simulink model "Filter_Fixed"  (R2017b)
settings: Solver=FixedStepDiscrete  StartTime=0.0  StopTime=400  RelTol=1e-3
undefined symbols (not defined in the file or in its folder): designMultirateFIR
libraries: dspmlti4 x1
(part 2 of 3)

== system Filter_Fixed/HighpassH/Resonator116 ==
  In1 : Inport
  Delay : Delay  DelayLength=1
  Gain : Gain  Gain=-0.67188-0.74066i  OutDataTypeStr=fixdt(1,24,23)
  GainH : Gain  Gain=0.39229-0.91984i  OutDataTypeStr=fixdt(1,24,23)
  Sum1 : Sum  Inputs=|++
  Out1 : Outport
  wires:
  In1/1 -> Sum1/1
  GainH/1 -> Out1/1
  Gain/1 -> Sum1/2
  Delay/1 -> Gain/1
  Sum1/1 -> Delay/1, GainH/1

== system Filter_Fixed/HighpassH/Resonator117 ==
  In1 : Inport
  Delay : Delay  DelayLength=1
  Gain : Gain  Gain=-0.65103-0.75905i  OutDataTypeStr=fixdt(1,24,23)
  GainH : Gain  Gain=-0.40504+0.9143i  OutDataTypeStr=fixdt(1,24,23)
  Sum1 : Sum  Inputs=|++
  Out1 : Outport
  wires:
  In1/1 -> Sum1/1
  GainH/1 -> Out1/1
  Gain/1 -> Sum1/2
  Delay/1 -> Gain/1
  Sum1/1 -> Delay/1, GainH/1

== system Filter_Fixed/HighpassH/Resonator118 ==
  In1 : Inport
  Delay : Delay  DelayLength=1
  Gain : Gain  Gain=-0.62968-0.77685i  OutDataTypeStr=fixdt(1,24,23)
  GainH : Gain  Gain=0.41771-0.90858i  OutDataTypeStr=fixdt(1,24,23)
  Sum1 : Sum  Inputs=|++
  Out1 : Outport
  wires:
  In1/1 -> Sum1/1
  GainH/1 -> Out1/1
  Gain/1 -> Sum1/2
  Delay/1 -> Gain/1
  Sum1/1 -> Delay/1, GainH/1

== system Filter_Fixed/HighpassH/Resonator119 ==
  In1 : Inport
  Delay : Delay  DelayLength=1
  Gain : Gain  Gain=-0.60784-0.79406i  OutDataTypeStr=fixdt(1,24,23)
  GainH : Gain  Gain=-0.4303+0.90269i  OutDataTypeStr=fixdt(1,24,23)
  Sum1 : Sum  Inputs=|++
  Out1 : Outport
  wires:
  In1/1 -> Sum1/1
  GainH/1 -> Out1/1
  Gain/1 -> Sum1/2
  Delay/1 -> Gain/1
  Sum1/1 -> Delay/1, GainH/1

== system Filter_Fixed/HighpassH/Resonator12 ==
  In1 : Inport
  Delay : Delay  DelayLength=1
  Gain : Gain  Gain=0.46756+0.88396i  OutDataTypeStr=fixdt(1,24,23)
  GainH : Gain  Gain=0.8637+0.50401i  OutDataTypeStr=fixdt(1,24,23)
  Sum1 : Sum  Inputs=|++
  Out1 : Outport
  wires:
  In1/1 -> Sum1/1
  GainH/1 -> Out1/1
  Gain/1 -> Sum1/2
  Delay/1 -> Gain/1
  Sum1/1 -> Delay/1, GainH/1

== system Filter_Fixed/HighpassH/Resonator120 ==
  In1 : Inport
  Delay : Delay  DelayLength=1
  Gain : Gain  Gain=-0.58553-0.81065i  OutDataTypeStr=fixdt(1,24,23)
  GainH : Gain  Gain=0.44281-0.89662i  OutDataTypeStr=fixdt(1,24,23)
  Sum1 : Sum  Inputs=|++
  Out1 : Outport
  wires:
  In1/1 -> Sum1/1
  GainH/1 -> Out1/1
  Gain/1 -> Sum1/2
  Delay/1 -> Gain/1
  Sum1/1 -> Delay/1, GainH/1

== system Filter_Fixed/HighpassH/Resonator121 ==
  In1 : Inport
  Delay : Delay  DelayLength=1
  Gain : Gain  Gain=-0.56277-0.82661i  OutDataTypeStr=fixdt(1,24,23)
  GainH : Gain  Gain=-0.45523+0.89037i  OutDataTypeStr=fixdt(1,24,23)
  Sum1 : Sum  Inputs=|++
  Out1 : Outport
  wires:
  In1/1 -> Sum1/1
  GainH/1 -> Out1/1
  Gain/1 -> Sum1/2
  Delay/1 -> Gain/1
  Sum1/1 -> Delay/1, GainH/1

== system Filter_Fixed/HighpassH/Resonator122 ==
  In1 : Inport
  Delay : Delay  DelayLength=1
  Gain : Gain  Gain=-0.53958-0.84194i  OutDataTypeStr=fixdt(1,24,23)
  GainH : Gain  Gain=0.46756-0.88396i  OutDataTypeStr=fixdt(1,24,23)
  Sum1 : Sum  Inputs=|++
  Out1 : Outport
  wires:
  In1/1 -> Sum1/1
  GainH/1 -> Out1/1
  Gain/1 -> Sum1/2
  Delay/1 -> Gain/1
  Sum1/1 -> Delay/1, GainH/1

== system Filter_Fixed/HighpassH/Resonator123 ==
  In1 : Inport
  Delay : Delay  DelayLength=1
  Gain : Gain  Gain=-0.51596-0.85661i  OutDataTypeStr=fixdt(1,24,23)
  GainH : Gain  Gain=-0.4798+0.87738i  OutDataTypeStr=fixdt(1,24,23)
  Sum1 : Sum  Inputs=|++
  Out1 : Outport
  wires:
  In1/1 -> Sum1/1
  GainH/1 -> Out1/1
  Gain/1 -> Sum1/2
  Delay/1 -> Gain/1
  Sum1/1 -> Delay/1, GainH/1

== system Filter_Fixed/HighpassH/Resonator124 ==
  In1 : Inport
  Delay : Delay  DelayLength=1
  Gain : Gain  Gain=-0.49195-0.87062i  OutDataTypeStr=fixdt(1,24,23)
  GainH : Gain  Gain=0.49195-0.87062i  OutDataTypeStr=fixdt(1,24,23)
  Sum1 : Sum  Inputs=|++
  Out1 : Outport
  wires:
  In1/1 -> Sum1/1
  GainH/1 -> Out1/1
  Gain/1 -> Sum1/2
  Delay/1 -> Gain/1
  Sum1/1 -> Delay/1, GainH/1

== system Filter_Fixed/HighpassH/Resonator125 ==
  In1 : Inport
  Delay : Delay  DelayLength=1
  Gain : Gain  Gain=-0.46756-0.88396i  OutDataTypeStr=fixdt(1,24,23)
  GainH : Gain  Gain=-0.50401+0.8637i  OutDataTypeStr=fixdt(1,24,23)
  Sum1 : Sum  Inputs=|++
  Out1 : Outport
  wires:
  In1/1 -> Sum1/1
  GainH/1 -> Out1/1
  Gain/1 -> Sum1/2
  Delay/1 -> Gain/1
  Sum1/1 -> Delay/1, GainH/1

== system Filter_Fixed/HighpassH/Resonator126 ==
  In1 : Inport
  Delay : Delay  DelayLength=1
  Gain : Gain  Gain=-0.44281-0.89662i  OutDataTypeStr=fixdt(1,24,23)
  GainH : Gain  Gain=0.51596-0.85661i  OutDataTypeStr=fixdt(1,24,23)
  Sum1 : Sum  Inputs=|++
  Out1 : Outport
  wires:
  In1/1 -> Sum1/1
  GainH/1 -> Out1/1
  Gain/1 -> Sum1/2
  Delay/1 -> Gain/1
  Sum1/1 -> Delay/1, GainH/1

== system Filter_Fixed/HighpassH/Resonator127 ==
  In1 : Inport
  Delay : Delay  DelayLength=1
  Gain : Gain  Gain=-0.41771-0.90858i  OutDataTypeStr=fixdt(1,24,23)
  GainH : Gain  Gain=-0.52782+0.84936i  OutDataTypeStr=fixdt(1,24,23)
  Sum1 : Sum  Inputs=|++
  Out1 : Outport
  wires:
  In1/1 -> Sum1/1
  GainH/1 -> Out1/1
  Gain/1 -> Sum1/2
  Delay/1 -> Gain/1
  Sum1/1 -> Delay/1, GainH/1

== system Filter_Fixed/HighpassH/Resonator128 ==
  In1 : Inport
  Delay : Delay  DelayLength=1
  Gain : Gain  Gain=-0.39229-0.91984i  OutDataTypeStr=fixdt(1,24,23)
  GainH : Gain  Gain=0.53958-0.84194i  OutDataTypeStr=fixdt(1,24,23)
  Sum1 : Sum  Inputs=|++
  Out1 : Outport
  wires:
  In1/1 -> Sum1/1
  GainH/1 -> Out1/1
  Gain/1 -> Sum1/2
  Delay/1 -> Gain/1
  Sum1/1 -> Delay/1, GainH/1

== system Filter_Fixed/HighpassH/Resonator129 ==
  In1 : Inport
  Delay : Delay  DelayLength=1
  Gain : Gain  Gain=-0.36657-0.93039i  OutDataTypeStr=fixdt(1,24,23)
  GainH : Gain  Gain=-0.55123+0.83435i  OutDataTypeStr=fixdt(1,24,23)
  Sum1 : Sum  Inputs=|++
  Out1 : Outport
  wires:
  In1/1 -> Sum1/1
  GainH/1 -> Out1/1
  Gain/1 -> Sum1/2
  Delay/1 -> Gain/1
  Sum1/1 -> Delay/1, GainH/1

== system Filter_Fixed/HighpassH/Resonator13 ==
  In1 : Inport
  Delay : Delay  DelayLength=1
  Gain : Gain  Gain=0.44281+0.89662i  OutDataTypeStr=fixdt(1,24,23)
  GainH : Gain  Gain=-0.85661-0.51596i  OutDataTypeStr=fixdt(1,24,23)
  Sum1 : Sum  Inputs=|++
  Out1 : Outport
  wires:
  In1/1 -> Sum1/1
  GainH/1 -> Out1/1
  Gain/1 -> Sum1/2
  Delay/1 -> Gain/1
  Sum1/1 -> Delay/1, GainH/1

== system Filter_Fixed/HighpassH/Resonator130 ==
  In1 : Inport
  Delay : Delay  DelayLength=1
  Gain : Gain  Gain=-0.34057-0.94022i  OutDataTypeStr=fixdt(1,24,23)
  GainH : Gain  Gain=0.56277-0.82661i  OutDataTypeStr=fixdt(1,24,23)
  Sum1 : Sum  Inputs=|++
  Out1 : Outport
  wires:
  In1/1 -> Sum1/1
  GainH/1 -> Out1/1
  Gain/1 -> Sum1/2
  Delay/1 -> Gain/1
  Sum1/1 -> Delay/1, GainH/1

== system Filter_Fixed/HighpassH/Resonator131 ==
  In1 : Inport
  Delay : Delay  DelayLength=1
  Gain : Gain  Gain=-0.3143-0.94932i  OutDataTypeStr=fixdt(1,24,23)
  GainH : Gain  Gain=-0.57421+0.81871i  OutDataTypeStr=fixdt(1,24,23)
  Sum1 : Sum  Inputs=|++
  Out1 : Outport
  wires:
  In1/1 -> Sum1/1
  GainH/1 -> Out1/1
  Gain/1 -> Sum1/2
  Delay/1 -> Gain/1
  Sum1/1 -> Delay/1, GainH/1

== system Filter_Fixed/HighpassH/Resonator132 ==
  In1 : Inport
  Delay : Delay  DelayLength=1
  Gain : Gain  Gain=-0.28779-0.95769i  OutDataTypeStr=fixdt(1,24,23)
  GainH : Gain  Gain=0.58553-0.81065i  OutDataTypeStr=fixdt(1,24,23)
  Sum1 : Sum  Inputs=|++
  Out1 : Outport
  wires:
  In1/1 -> Sum1/1
  GainH/1 -> Out1/1
  Gain/1 -> Sum1/2
  Delay/1 -> Gain/1
  Sum1/1 -> Delay/1, GainH/1

== system Filter_Fixed/HighpassH/Resonator133 ==
  In1 : Inport
  Delay : Delay  DelayLength=1
  Gain : Gain  Gain=-0.26106-0.96532i  OutDataTypeStr=fixdt(1,24,23)
  GainH : Gain  Gain=-0.59675+0.80243i  OutDataTypeStr=fixdt(1,24,23)
  Sum1 : Sum  Inputs=|++
  Out1 : Outport
  wires:
  In1/1 -> Sum1/1
  GainH/1 -> Out1/1
  Gain/1 -> Sum1/2
  Delay/1 -> Gain/1
  Sum1/1 -> Delay/1, GainH/1

== system Filter_Fixed/HighpassH/Resonator134 ==
  In1 : Inport
  Delay : Delay  DelayLength=1
  Gain : Gain  Gain=-0.23412-0.97221i  OutDataTypeStr=fixdt(1,24,23)
  GainH : Gain  Gain=0.60784-0.79406i  OutDataTypeStr=fixdt(1,24,23)
  Sum1 : Sum  Inputs=|++
  Out1 : Outport
  wires:
  In1/1 -> Sum1/1
  GainH/1 -> Out1/1
  Gain/1 -> Sum1/2
  Delay/1 -> Gain/1
  Sum1/1 -> Delay/1, GainH/1

== system Filter_Fixed/HighpassH/Resonator135 ==
  In1 : Inport
  Delay : Delay  DelayLength=1
  Gain : Gain  Gain=-0.20701-0.97834i  OutDataTypeStr=fixdt(1,24,23)
  GainH : Gain  Gain=-0.61882+0.78553i  OutDataTypeStr=fixdt(1,24,23)
  Sum1 : Sum  Inputs=|++
  Out1 : Outport
  wires:
  In1/1 -> Sum1/1
  GainH/1 -> Out1/1
  Gain/1 -> Sum1/2
  Delay/1 -> Gain/1
  Sum1/1 -> Delay/1, GainH/1

== system Filter_Fixed/HighpassH/Resonator136 ==
  In1 : Inport
  Delay : Delay  DelayLength=1
  Gain : Gain  Gain=-0.17973-0.98372i  OutDataTypeStr=fixdt(1,24,23)
  GainH : Gain  Gain=0.62968-0.77685i  OutDataTypeStr=fixdt(1,24,23)
  Sum1 : Sum  Inputs=|++
  Out1 : Outport
  wires:
  In1/1 -> Sum1/1
  GainH/1 -> Out1/1
  Gain/1 -> Sum1/2
  Delay/1 -> Gain/1
  Sum1/1 -> Delay/1, GainH/1

== system Filter_Fixed/HighpassH/Resonator137 ==
  In1 : Inport
  Delay : Delay  DelayLength=1
  Gain : Gain  Gain=-0.15231-0.98833i  OutDataTypeStr=fixdt(1,24,23)
  GainH : Gain  Gain=-0.64042+0.76803i  OutDataTypeStr=fixdt(1,24,23)
  Sum1 : Sum  Inputs=|++
  Out1 : Outport
  wires:
  In1/1 -> Sum1/1
  GainH/1 -> Out1/1
  Gain/1 -> Sum1/2
  Delay/1 -> Gain/1
  Sum1/1 -> Delay/1, GainH/1

== system Filter_Fixed/HighpassH/Resonator138 ==
  In1 : Inport
  Delay : Delay  DelayLength=1
  Gain : Gain  Gain=-0.12478-0.99218i  OutDataTypeStr=fixdt(1,24,23)
  GainH : Gain  Gain=0.65103-0.75905i  OutDataTypeStr=fixdt(1,24,23)
  Sum1 : Sum  Inputs=|++
  Out1 : Outport
  wires:
  In1/1 -> Sum1/1
  GainH/1 -> Out1/1
  Gain/1 -> Sum1/2
  Delay/1 -> Gain/1
  Sum1/1 -> Delay/1, GainH/1

== system Filter_Fixed/HighpassH/Resonator139 ==
  In1 : Inport
  Delay : Delay  DelayLength=1
  Gain : Gain  Gain=-0.097152-0.99527i  OutDataTypeStr=fixdt(1,24,23)
  GainH : Gain  Gain=-0.66152+0.74993i  OutDataTypeStr=fixdt(1,24,23)
  Sum1 : Sum  Inputs=|++
  Out1 : Outport
  wires:
  In1/1 -> Sum1/1
  GainH/1 -> Out1/1
  Gain/1 -> Sum1/2
  Delay/1 -> Gain/1
  Sum1/1 -> Delay/1, GainH/1

== system Filter_Fixed/HighpassH/Resonator14 ==
  In1 : Inport
  Delay : Delay  DelayLength=1
  Gain : Gain  Gain=0.41771+0.90858i  OutDataTypeStr=fixdt(1,24,23)
  GainH : Gain  Gain=0.84936+0.52782i  OutDataTypeStr=fixdt(1,24,23)
  Sum1 : Sum  Inputs=|++
  Out1 : Outport
  wires:
  In1/1 -> Sum1/1
  GainH/1 -> Out1/1
  Gain/1 -> Sum1/2
  Delay/1 -> Gain/1
  Sum1/1 -> Delay/1, GainH/1

== system Filter_Fixed/HighpassH/Resonator140 ==
  In1 : Inport
  Delay : Delay  DelayLength=1
  Gain : Gain  Gain=-0.069448-0.99759i  OutDataTypeStr=fixdt(1,24,23)
  GainH : Gain  Gain=0.67188-0.74066i  OutDataTypeStr=fixdt(1,24,23)
  Sum1 : Sum  Inputs=|++
  Out1 : Outport
  wires:
  In1/1 -> Sum1/1
  GainH/1 -> Out1/1
  Gain/1 -> Sum1/2
  Delay/1 -> Gain/1
  Sum1/1 -> Delay/1, GainH/1

== system Filter_Fixed/HighpassH/Resonator141 ==
  In1 : Inport
  Delay : Delay  DelayLength=1
  Gain : Gain  Gain=-0.04169-0.99913i  OutDataTypeStr=fixdt(1,24,23)
  GainH : Gain  Gain=-0.68211+0.73125i  OutDataTypeStr=fixdt(1,24,23)
  Sum1 : Sum  Inputs=|++
  Out1 : Outport
  wires:
  In1/1 -> Sum1/1
  GainH/1 -> Out1/1
  Gain/1 -> Sum1/2
  Delay/1 -> Gain/1
  Sum1/1 -> Delay/1, GainH/1

== system Filter_Fixed/HighpassH/Resonator142 ==
  In1 : Inport
  Delay : Delay  DelayLength=1
  Gain : Gain  Gain=-0.0139-0.9999i  OutDataTypeStr=fixdt(1,24,23)
  GainH : Gain  Gain=0.69221-0.7217i  OutDataTypeStr=fixdt(1,24,23)
  Sum1 : Sum  Inputs=|++
  Out1 : Outport
  wires:
  In1/1 -> Sum1/1
  GainH/1 -> Out1/1
  Gain/1 -> Sum1/2
  Delay/1 -> Gain/1
  Sum1/1 -> Delay/1, GainH/1

== system Filter_Fixed/HighpassH/Resonator143 ==
  In1 : Inport
  Delay : Delay  DelayLength=1
  Gain : Gain  Gain=0.0139-0.9999i  OutDataTypeStr=fixdt(1,24,23)
  GainH : Gain  Gain=-0.70218+0.712i  OutDataTypeStr=fixdt(1,24,23)
  Sum1 : Sum  Inputs=|++
  Out1 : Outport
  wires:
  In1/1 -> Sum1/1
  GainH/1 -> Out1/1
  Gain/1 -> Sum1/2
  Delay/1 -> Gain/1
  Sum1/1 -> Delay/1, GainH/1

== system Filter_Fixed/HighpassH/Resonator144 ==
  In1 : Inport
  Delay : Delay  DelayLength=1
  Gain : Gain  Gain=0.04169-0.99913i  OutDataTypeStr=fixdt(1,24,23)
  GainH : Gain  Gain=0.712-0.70218i  OutDataTypeStr=fixdt(1,24,23)
  Sum1 : Sum  Inputs=|++
  Out1 : Outport
  wires:
  In1/1 -> Sum1/1
  GainH/1 -> Out1/1
  Gain/1 -> Sum1/2
  Delay/1 -> Gain/1
  Sum1/1 -> Delay/1, GainH/1

== system Filter_Fixed/HighpassH/Resonator145 ==
  In1 : Inport
  Delay : Delay  DelayLength=1
  Gain : Gain  Gain=0.069448-0.99759i  OutDataTypeStr=fixdt(1,24,23)
  GainH : Gain  Gain=-0.7217+0.69221i  OutDataTypeStr=fixdt(1,24,23)
  Sum1 : Sum  Inputs=|++
  Out1 : Outport
  wires:
  In1/1 -> Sum1/1
  GainH/1 -> Out1/1
  Gain/1 -> Sum1/2
  Delay/1 -> Gain/1
  Sum1/1 -> Delay/1, GainH/1

== system Filter_Fixed/HighpassH/Resonator146 ==
  In1 : Inport
  Delay : Delay  DelayLength=1
  Gain : Gain  Gain=0.097152-0.99527i  OutDataTypeStr=fixdt(1,24,23)
  GainH : Gain  Gain=0.73125-0.68211i  OutDataTypeStr=fixdt(1,24,23)
  Sum1 : Sum  Inputs=|++
  Out1 : Outport
  wires:
  In1/1 -> Sum1/1
  GainH/1 -> Out1/1
  Gain/1 -> Sum1/2
  Delay/1 -> Gain/1
  Sum1/1 -> Delay/1, GainH/1

== system Filter_Fixed/HighpassH/Resonator147 ==
  In1 : Inport
  Delay : Delay  DelayLength=1
  Gain : Gain  Gain=0.12478-0.99218i  OutDataTypeStr=fixdt(1,24,23)
  GainH : Gain  Gain=-0.74066+0.67188i  OutDataTypeStr=fixdt(1,24,23)
  Sum1 : Sum  Inputs=|++
  Out1 : Outport
  wires:
  In1/1 -> Sum1/1
  GainH/1 -> Out1/1
  Gain/1 -> Sum1/2
  Delay/1 -> Gain/1
  Sum1/1 -> Delay/1, GainH/1

== system Filter_Fixed/HighpassH/Resonator148 ==
  In1 : Inport
  Delay : Delay  DelayLength=1
  Gain : Gain  Gain=0.15231-0.98833i  OutDataTypeStr=fixdt(1,24,23)
  GainH : Gain  Gain=0.74993-0.66152i  OutDataTypeStr=fixdt(1,24,23)
  Sum1 : Sum  Inputs=|++
  Out1 : Outport
  wires:
  In1/1 -> Sum1/1
  GainH/1 -> Out1/1
  Gain/1 -> Sum1/2
  Delay/1 -> Gain/1
  Sum1/1 -> Delay/1, GainH/1

== system Filter_Fixed/HighpassH/Resonator149 ==
  In1 : Inport
  Delay : Delay  DelayLength=1
  Gain : Gain  Gain=0.17973-0.98372i  OutDataTypeStr=fixdt(1,24,23)
  GainH : Gain  Gain=-0.75905+0.65103i  OutDataTypeStr=fixdt(1,24,23)
  Sum1 : Sum  Inputs=|++
  Out1 : Outport
  wires:
  In1/1 -> Sum1/1
  GainH/1 -> Out1/1
  Gain/1 -> Sum1/2
  Delay/1 -> Gain/1
  Sum1/1 -> Delay/1, GainH/1

== system Filter_Fixed/HighpassH/Resonator15 ==
  In1 : Inport
  Delay : Delay  DelayLength=1
  Gain : Gain  Gain=0.39229+0.91984i  OutDataTypeStr=fixdt(1,24,23)
  GainH : Gain  Gain=-0.84194-0.53958i  OutDataTypeStr=fixdt(1,24,23)
  Sum1 : Sum  Inputs=|++
  Out1 : Outport
  wires:
  In1/1 -> Sum1/1
  GainH/1 -> Out1/1
  Gain/1 -> Sum1/2
  Delay/1 -> Gain/1
  Sum1/1 -> Delay/1, GainH/1

== system Filter_Fixed/HighpassH/Resonator150 ==
  In1 : Inport
  Delay : Delay  DelayLength=1
  Gain : Gain  Gain=0.20701-0.97834i  OutDataTypeStr=fixdt(1,24,23)
  GainH : Gain  Gain=0.76803-0.64042i  OutDataTypeStr=fixdt(1,24,23)
  Sum1 : Sum  Inputs=|++
  Out1 : Outport
  wires:
  In1/1 -> Sum1/1
  GainH/1 -> Out1/1
  Gain/1 -> Sum1/2
  Delay/1 -> Gain/1
  Sum1/1 -> Delay/1, GainH/1

== system Filter_Fixed/HighpassH/Resonator151 ==
  In1 : Inport
  Delay : Delay  DelayLength=1
  Gain : Gain  Gain=0.23412-0.97221i  OutDataTypeStr=fixdt(1,24,23)
  GainH : Gain  Gain=-0.77685+0.62968i  OutDataTypeStr=fixdt(1,24,23)
  Sum1 : Sum  Inputs=|++
  Out1 : Outport
  wires:
  In1/1 -> Sum1/1
  GainH/1 -> Out1/1
  Gain/1 -> Sum1/2
  Delay/1 -> Gain/1
  Sum1/1 -> Delay/1, GainH/1

== system Filter_Fixed/HighpassH/Resonator152 ==
  In1 : Inport
  Delay : Delay  DelayLength=1
  Gain : Gain  Gain=0.26106-0.96532i  OutDataTypeStr=fixdt(1,24,23)
  GainH : Gain  Gain=0.78553-0.61882i  OutDataTypeStr=fixdt(1,24,23)
  Sum1 : Sum  Inputs=|++
  Out1 : Outport
  wires:
  In1/1 -> Sum1/1
  GainH/1 -> Out1/1
  Gain/1 -> Sum1/2
  Delay/1 -> Gain/1
  Sum1/1 -> Delay/1, GainH/1

== system Filter_Fixed/HighpassH/Resonator153 ==
  In1 : Inport
  Delay : Delay  DelayLength=1
  Gain : Gain  Gain=0.28779-0.95769i  OutDataTypeStr=fixdt(1,24,23)
  GainH : Gain  Gain=-0.79406+0.60784i  OutDataTypeStr=fixdt(1,24,23)
  Sum1 : Sum  Inputs=|++
  Out1 : Outport
  wires:
  In1/1 -> Sum1/1
  GainH/1 -> Out1/1
  Gain/1 -> Sum1/2
  Delay/1 -> Gain/1
  Sum1/1 -> Delay/1, GainH/1

== system Filter_Fixed/HighpassH/Resonator154 ==
  In1 : Inport
  Delay : Delay  DelayLength=1
  Gain : Gain  Gain=0.3143-0.94932i  OutDataTypeStr=fixdt(1,24,23)
  GainH : Gain  Gain=0.80243-0.59675i  OutDataTypeStr=fixdt(1,24,23)
  Sum1 : Sum  Inputs=|++
  Out1 : Outport
  wires:
  In1/1 -> Sum1/1
  GainH/1 -> Out1/1
  Gain/1 -> Sum1/2
  Delay/1 -> Gain/1
  Sum1/1 -> Delay/1, GainH/1

== system Filter_Fixed/HighpassH/Resonator155 ==
  In1 : Inport
  Delay : Delay  DelayLength=1
  Gain : Gain  Gain=0.34057-0.94022i  OutDataTypeStr=fixdt(1,24,23)
  GainH : Gain  Gain=-0.81065+0.58553i  OutDataTypeStr=fixdt(1,24,23)
  Sum1 : Sum  Inputs=|++
  Out1 : Outport
  wires:
  In1/1 -> Sum1/1
  GainH/1 -> Out1/1
  Gain/1 -> Sum1/2
  Delay/1 -> Gain/1
  Sum1/1 -> Delay/1, GainH/1

== system Filter_Fixed/HighpassH/Resonator156 ==
  In1 : Inport
  Delay : Delay  DelayLength=1
  Gain : Gain  Gain=0.36657-0.93039i  OutDataTypeStr=fixdt(1,24,23)
  GainH : Gain  Gain=0.81871-0.57421i  OutDataTypeStr=fixdt(1,24,23)
  Sum1 : Sum  Inputs=|++
  Out1 : Outport
  wires:
  In1/1 -> Sum1/1
  GainH/1 -> Out1/1
  Gain/1 -> Sum1/2
  Delay/1 -> Gain/1
  Sum1/1 -> Delay/1, GainH/1

== system Filter_Fixed/HighpassH/Resonator157 ==
  In1 : Inport
  Delay : Delay  DelayLength=1
  Gain : Gain  Gain=0.39229-0.91984i  OutDataTypeStr=fixdt(1,24,23)
  GainH : Gain  Gain=-0.82661+0.56277i  OutDataTypeStr=fixdt(1,24,23)
  Sum1 : Sum  Inputs=|++
  Out1 : Outport
  wires:
  In1/1 -> Sum1/1
  GainH/1 -> Out1/1
  Gain/1 -> Sum1/2
  Delay/1 -> Gain/1
  Sum1/1 -> Delay/1, GainH/1

== system Filter_Fixed/HighpassH/Resonator158 ==
  In1 : Inport
  Delay : Delay  DelayLength=1
  Gain : Gain  Gain=0.41771-0.90858i  OutDataTypeStr=fixdt(1,24,23)
  GainH : Gain  Gain=0.83435-0.55123i  OutDataTypeStr=fixdt(1,24,23)
  Sum1 : Sum  Inputs=|++
  Out1 : Outport
  wires:
  In1/1 -> Sum1/1
  GainH/1 -> Out1/1
  Gain/1 -> Sum1/2
  Delay/1 -> Gain/1
  Sum1/1 -> Delay/1, GainH/1

== system Filter_Fixed/HighpassH/Resonator159 ==
  In1 : Inport
  Delay : Delay  DelayLength=1
  Gain : Gain  Gain=0.44281-0.89662i  OutDataTypeStr=fixdt(1,24,23)
  GainH : Gain  Gain=-0.84194+0.53958i  OutDataTypeStr=fixdt(1,24,23)
  Sum1 : Sum  Inputs=|++
  Out1 : Outport
  wires:
  In1/1 -> Sum1/1
  GainH/1 -> Out1/1
  Gain/1 -> Sum1/2
  Delay/1 -> Gain/1
  Sum1/1 -> Delay/1, GainH/1

== system Filter_Fixed/HighpassH/Resonator16 ==
  In1 : Inport
  Delay : Delay  DelayLength=1
  Gain : Gain  Gain=0.36657+0.93039i  OutDataTypeStr=fixdt(1,24,23)
  GainH : Gain  Gain=0.83435+0.55123i  OutDataTypeStr=fixdt(1,24,23)
  Sum1 : Sum  Inputs=|++
  Out1 : Outport
  wires:
  In1/1 -> Sum1/1
  GainH/1 -> Out1/1
  Gain/1 -> Sum1/2
  Delay/1 -> Gain/1
  Sum1/1 -> Delay/1, GainH/1

== system Filter_Fixed/HighpassH/Resonator160 ==
  In1 : Inport
  Delay : Delay  DelayLength=1
  Gain : Gain  Gain=0.46756-0.88396i  OutDataTypeStr=fixdt(1,24,23)
  GainH : Gain  Gain=0.84936-0.52782i  OutDataTypeStr=fixdt(1,24,23)
  Sum1 : Sum  Inputs=|++
  Out1 : Outport
  wires:
  In1/1 -> Sum1/1
  GainH/1 -> Out1/1
  Gain/1 -> Sum1/2
  Delay/1 -> Gain/1
  Sum1/1 -> Delay/1, GainH/1

== system Filter_Fixed/HighpassH/Resonator161 ==
  In1 : Inport
  Delay : Delay  DelayLength=1
  Gain : Gain  Gain=0.49195-0.87062i  OutDataTypeStr=fixdt(1,24,23)
  GainH : Gain  Gain=-0.85661+0.51596i  OutDataTypeStr=fixdt(1,24,23)
  Sum1 : Sum  Inputs=|++
  Out1 : Outport
  wires:
  In1/1 -> Sum1/1
  GainH/1 -> Out1/1
  Gain/1 -> Sum1/2
  Delay/1 -> Gain/1
  Sum1/1 -> Delay/1, GainH/1

== system Filter_Fixed/HighpassH/Resonator162 ==
  In1 : Inport
  Delay : Delay  DelayLength=1
  Gain : Gain  Gain=0.51596-0.85661i  OutDataTypeStr=fixdt(1,24,23)
  GainH : Gain  Gain=0.8637-0.50401i  OutDataTypeStr=fixdt(1,24,23)
  Sum1 : Sum  Inputs=|++
  Out1 : Outport
  wires:
  In1/1 -> Sum1/1
  GainH/1 -> Out1/1
  Gain/1 -> Sum1/2
  Delay/1 -> Gain/1
  Sum1/1 -> Delay/1, GainH/1

== system Filter_Fixed/HighpassH/Resonator163 ==
  In1 : Inport
  Delay : Delay  DelayLength=1
  Gain : Gain  Gain=0.53958-0.84194i  OutDataTypeStr=fixdt(1,24,23)
  GainH : Gain  Gain=-0.87062+0.49195i  OutDataTypeStr=fixdt(1,24,23)
  Sum1 : Sum  Inputs=|++
  Out1 : Outport
  wires:
  In1/1 -> Sum1/1
  GainH/1 -> Out1/1
  Gain/1 -> Sum1/2
  Delay/1 -> Gain/1
  Sum1/1 -> Delay/1, GainH/1

== system Filter_Fixed/HighpassH/Resonator164 ==
  In1 : Inport
  Delay : Delay  DelayLength=1
  Gain : Gain  Gain=0.56277-0.82661i  OutDataTypeStr=fixdt(1,24,23)
  GainH : Gain  Gain=0.87738-0.4798i  OutDataTypeStr=fixdt(1,24,23)
  Sum1 : Sum  Inputs=|++
  Out1 : Outport
  wires:
  In1/1 -> Sum1/1
  GainH/1 -> Out1/1
  Gain/1 -> Sum1/2
  Delay/1 -> Gain/1
  Sum1/1 -> Delay/1, GainH/1

== system Filter_Fixed/HighpassH/Resonator165 ==
  In1 : Inport
  Delay : Delay  DelayLength=1
  Gain : Gain  Gain=0.58553-0.81065i  OutDataTypeStr=fixdt(1,24,23)
  GainH : Gain  Gain=-0.88396+0.46756i  OutDataTypeStr=fixdt(1,24,23)
  Sum1 : Sum  Inputs=|++
  Out1 : Outport
  wires:
  In1/1 -> Sum1/1
  GainH/1 -> Out1/1
  Gain/1 -> Sum1/2
  Delay/1 -> Gain/1
  Sum1/1 -> Delay/1, GainH/1

== system Filter_Fixed/HighpassH/Resonator166 ==
  In1 : Inport
  Delay : Delay  DelayLength=1
  Gain : Gain  Gain=0.60784-0.79406i  OutDataTypeStr=fixdt(1,24,23)
  GainH : Gain  Gain=0.89037-0.45523i  OutDataTypeStr=fixdt(1,24,23)
  Sum1 : Sum  Inputs=|++
  Out1 : Outport
  wires:
  In1/1 -> Sum1/1
  GainH/1 -> Out1/1
  Gain/1 -> Sum1/2
  Delay/1 -> Gain/1
  Sum1/1 -> Delay/1, GainH/1

== system Filter_Fixed/HighpassH/Resonator167 ==
  In1 : Inport
  Delay : Delay  DelayLength=1
  Gain : Gain  Gain=0.62968-0.77685i  OutDataTypeStr=fixdt(1,24,23)
  GainH : Gain  Gain=-0.89662+0.44281i  OutDataTypeStr=fixdt(1,24,23)
  Sum1 : Sum  Inputs=|++
  Out1 : Outport
  wires:
  In1/1 -> Sum1/1
  GainH/1 -> Out1/1
  Gain/1 -> Sum1/2
  Delay/1 -> Gain/1
  Sum1/1 -> Delay/1, GainH/1

== system Filter_Fixed/HighpassH/Resonator168 ==
  In1 : Inport
  Delay : Delay  DelayLength=1
  Gain : Gain  Gain=0.65103-0.75905i  OutDataTypeStr=fixdt(1,24,23)
  GainH : Gain  Gain=0.90269-0.4303i  OutDataTypeStr=fixdt(1,24,23)
  Sum1 : Sum  Inputs=|++
  Out1 : Outport
  wires:
  In1/1 -> Sum1/1
  GainH/1 -> Out1/1
  Gain/1 -> Sum1/2
  Delay/1 -> Gain/1
  Sum1/1 -> Delay/1, GainH/1

== system Filter_Fixed/HighpassH/Resonator169 ==
  In1 : Inport
  Delay : Delay  DelayLength=1
  Gain : Gain  Gain=0.67188-0.74066i  OutDataTypeStr=fixdt(1,24,23)
  GainH : Gain  Gain=-0.90858+0.41771i  OutDataTypeStr=fixdt(1,24,23)
  Sum1 : Sum  Inputs=|++
  Out1 : Outport
  wires:
  In1/1 -> Sum1/1
  GainH/1 -> Out1/1
  Gain/1 -> Sum1/2
  Delay/1 -> Gain/1
  Sum1/1 -> Delay/1, GainH/1

== system Filter_Fixed/HighpassH/Resonator17 ==
  In1 : Inport
  Delay : Delay  DelayLength=1
  Gain : Gain  Gain=0.34057+0.94022i  OutDataTypeStr=fixdt(1,24,23)
  GainH : Gain  Gain=-0.82661-0.56277i  OutDataTypeStr=fixdt(1,24,23)
  Sum1 : Sum  Inputs=|++
  Out1 : Outport
  wires:
  In1/1 -> Sum1/1
  GainH/1 -> Out1/1
  Gain/1 -> Sum1/2
  Delay/1 -> Gain/1
  Sum1/1 -> Delay/1, GainH/1

== system Filter_Fixed/HighpassH/Resonator170 ==
  In1 : Inport
  Delay : Delay  DelayLength=1
  Gain : Gain  Gain=0.69221-0.7217i  OutDataTypeStr=fixdt(1,24,23)
  GainH : Gain  Gain=0.9143-0.40504i  OutDataTypeStr=fixdt(1,24,23)
  Sum1 : Sum  Inputs=|++
  Out1 : Outport
  wires:
  In1/1 -> Sum1/1
  GainH/1 -> Out1/1
  Gain/1 -> Sum1/2
  Delay/1 -> Gain/1
  Sum1/1 -> Delay/1, GainH/1

== system Filter_Fixed/HighpassH/Resonator171 ==
  In1 : Inport
  Delay : Delay  DelayLength=1
  Gain : Gain  Gain=0.712-0.70218i  OutDataTypeStr=fixdt(1,24,23)
  GainH : Gain  Gain=-0.91984+0.39229i  OutDataTypeStr=fixdt(1,24,23)
  Sum1 : Sum  Inputs=|++
  Out1 : Outport
  wires:
  In1/1 -> Sum1/1
  GainH/1 -> Out1/1
  Gain/1 -> Sum1/2
  Delay/1 -> Gain/1
  Sum1/1 -> Delay/1, GainH/1

== system Filter_Fixed/HighpassH/Resonator172 ==
  In1 : Inport
  Delay : Delay  DelayLength=1
  Gain : Gain  Gain=0.73125-0.68211i  OutDataTypeStr=fixdt(1,24,23)
  GainH : Gain  Gain=0.9252-0.37947i  OutDataTypeStr=fixdt(1,24,23)
  Sum1 : Sum  Inputs=|++
  Out1 : Outport
  wires:
  In1/1 -> Sum1/1
  GainH/1 -> Out1/1
  Gain/1 -> Sum1/2
  Delay/1 -> Gain/1
  Sum1/1 -> Delay/1, GainH/1

== system Filter_Fixed/HighpassH/Resonator173 ==
  In1 : Inport
  Delay : Delay  DelayLength=1
  Gain : Gain  Gain=0.74993-0.66152i  OutDataTypeStr=fixdt(1,24,23)
  GainH : Gain  Gain=-0.93039+0.36657i  OutDataTypeStr=fixdt(1,24,23)
  Sum1 : Sum  Inputs=|++
  Out1 : Outport
  wires:
  In1/1 -> Sum1/1
  GainH/1 -> Out1/1
  Gain/1 -> Sum1/2
  Delay/1 -> Gain/1
  Sum1/1 -> Delay/1, GainH/1

== system Filter_Fixed/HighpassH/Resonator18 ==
  In1 : Inport
  Delay : Delay  DelayLength=1
  Gain : Gain  Gain=0.3143+0.94932i  OutDataTypeStr=fixdt(1,24,23)
  GainH : Gain  Gain=0.81871+0.57421i  OutDataTypeStr=fixdt(1,24,23)
  Sum1 : Sum  Inputs=|++
  Out1 : Outport
  wires:
  In1/1 -> Sum1/1
  GainH/1 -> Out1/1
  Gain/1 -> Sum1/2
  Delay/1 -> Gain/1
  Sum1/1 -> Delay/1, GainH/1

== system Filter_Fixed/HighpassH/Resonator19 ==
  In1 : Inport
  Delay : Delay  DelayLength=1
  Gain : Gain  Gain=0.28779+0.95769i  OutDataTypeStr=fixdt(1,24,23)
  GainH : Gain  Gain=-0.81065-0.58553i  OutDataTypeStr=fixdt(1,24,23)
  Sum1 : Sum  Inputs=|++
  Out1 : Outport
  wires:
  In1/1 -> Sum1/1
  GainH/1 -> Out1/1
  Gain/1 -> Sum1/2
  Delay/1 -> Gain/1
  Sum1/1 -> Delay/1, GainH/1

== system Filter_Fixed/HighpassH/Resonator2 ==
  In1 : Inport
  Delay : Delay  DelayLength=1
  Gain : Gain  Gain=0.69221+0.7217i  OutDataTypeStr=fixdt(1,24,23)
  GainH : Gain  Gain=0.9252+0.37947i  OutDataTypeStr=fixdt(1,24,23)
  Sum1 : Sum  Inputs=|++
  Out1 : Outport
  wires:
  In1/1 -> Sum1/1
  GainH/1 -> Out1/1
  Gain/1 -> Sum1/2
  Delay/1 -> Gain/1
  Sum1/1 -> Delay/1, GainH/1

== system Filter_Fixed/HighpassH/Resonator20 ==
  In1 : Inport
  Delay : Delay  DelayLength=1
  Gain : Gain  Gain=0.26106+0.96532i  OutDataTypeStr=fixdt(1,24,23)
  GainH : Gain  Gain=0.80243+0.59675i  OutDataTypeStr=fixdt(1,24,23)
  Sum1 : Sum  Inputs=|++
  Out1 : Outport
  wires:
  In1/1 -> Sum1/1
  GainH/1 -> Out1/1
  Gain/1 -> Sum1/2
  Delay/1 -> Gain/1
  Sum1/1 -> Delay/1, GainH/1

== system Filter_Fixed/HighpassH/Resonator21 ==
  In1 : Inport
  Delay : Delay  DelayLength=1
  Gain : Gain  Gain=0.23412+0.97221i  OutDataTypeStr=fixdt(1,24,23)
  GainH : Gain  Gain=-0.79406-0.60784i  OutDataTypeStr=fixdt(1,24,23)
  Sum1 : Sum  Inputs=|++
  Out1 : Outport
  wires:
  In1/1 -> Sum1/1
  GainH/1 -> Out1/1
  Gain/1 -> Sum1/2
  Delay/1 -> Gain/1
  Sum1/1 -> Delay/1, GainH/1

== system Filter_Fixed/HighpassH/Resonator22 ==
  In1 : Inport
  Delay : Delay  DelayLength=1
  Gain : Gain  Gain=0.20701+0.97834i  OutDataTypeStr=fixdt(1,24,23)
  GainH : Gain  Gain=0.78553+0.61882i  OutDataTypeStr=fixdt(1,24,23)
  Sum1 : Sum  Inputs=|++
  Out1 : Outport
  wires:
  In1/1 -> Sum1/1
  GainH/1 -> Out1/1
  Gain/1 -> Sum1/2
  Delay/1 -> Gain/1
  Sum1/1 -> Delay/1, GainH/1

== system Filter_Fixed/HighpassH/Resonator23 ==
  In1 : Inport
  Delay : Delay  DelayLength=1
  Gain : Gain  Gain=0.17973+0.98372i  OutDataTypeStr=fixdt(1,24,23)
  GainH : Gain  Gain=-0.77685-0.62968i  OutDataTypeStr=fixdt(1,24,23)
  Sum1 : Sum  Inputs=|++
  Out1 : Outport
  wires:
  In1/1 -> Sum1/1
  GainH/1 -> Out1/1
  Gain/1 -> Sum1/2
  Delay/1 -> Gain/1
  Sum1/1 -> Delay/1, GainH/1

== system Filter_Fixed/HighpassH/Resonator24 ==
  In1 : Inport
  Delay : Delay  DelayLength=1
  Gain : Gain  Gain=0.15231+0.98833i  OutDataTypeStr=fixdt(1,24,23)
  GainH : Gain  Gain=0.76803+0.64042i  OutDataTypeStr=fixdt(1,24,23)
  Sum1 : Sum  Inputs=|++
  Out1 : Outport
  wires:
  In1/1 -> Sum1/1
  GainH/1 -> Out1/1
  Gain/1 -> Sum1/2
  Delay/1 -> Gain/1
  Sum1/1 -> Delay/1, GainH/1

== system Filter_Fixed/HighpassH/Resonator25 ==
  In1 : Inport
  Delay : Delay  DelayLength=1
  Gain : Gain  Gain=0.12478+0.99218i  OutDataTypeStr=fixdt(1,24,23)
  GainH : Gain  Gain=-0.75905-0.65103i  OutDataTypeStr=fixdt(1,24,23)
  Sum1 : Sum  Inputs=|++
  Out1 : Outport
  wires:
  In1/1 -> Sum1/1
  GainH/1 -> Out1/1
  Gain/1 -> Sum1/2
  Delay/1 -> Gain/1
  Sum1/1 -> Delay/1, GainH/1

== system Filter_Fixed/HighpassH/Resonator26 ==
  In1 : Inport
  Delay : Delay  DelayLength=1
  Gain : Gain  Gain=0.097152+0.99527i  OutDataTypeStr=fixdt(1,24,23)
  GainH : Gain  Gain=0.74993+0.66152i  OutDataTypeStr=fixdt(1,24,23)
  Sum1 : Sum  Inputs=|++
  Out1 : Outport
  wires:
  In1/1 -> Sum1/1
  GainH/1 -> Out1/1
  Gain/1 -> Sum1/2
  Delay/1 -> Gain/1
  Sum1/1 -> Delay/1, GainH/1

== system Filter_Fixed/HighpassH/Resonator27 ==
  In1 : Inport
  Delay : Delay  DelayLength=1
  Gain : Gain  Gain=0.069448+0.99759i  OutDataTypeStr=fixdt(1,24,23)
  GainH : Gain  Gain=-0.74066-0.67188i  OutDataTypeStr=fixdt(1,24,23)
  Sum1 : Sum  Inputs=|++
  Out1 : Outport
  wires:
  In1/1 -> Sum1/1
  GainH/1 -> Out1/1
  Gain/1 -> Sum1/2
  Delay/1 -> Gain/1
  Sum1/1 -> Delay/1, GainH/1

== system Filter_Fixed/HighpassH/Resonator28 ==
  In1 : Inport
  Delay : Delay  DelayLength=1
  Gain : Gain  Gain=0.04169+0.99913i  OutDataTypeStr=fixdt(1,24,23)
  GainH : Gain  Gain=0.73125+0.68211i  OutDataTypeStr=fixdt(1,24,23)
  Sum1 : Sum  Inputs=|++
  Out1 : Outport
  wires:
  In1/1 -> Sum1/1
  GainH/1 -> Out1/1
  Gain/1 -> Sum1/2
  Delay/1 -> Gain/1
  Sum1/1 -> Delay/1, GainH/1

== system Filter_Fixed/HighpassH/Resonator29 ==
  In1 : Inport
  Delay : Delay  DelayLength=1
  Gain : Gain  Gain=0.0139+0.9999i  OutDataTypeStr=fixdt(1,24,23)
  GainH : Gain  Gain=-0.7217-0.69221i  OutDataTypeStr=fixdt(1,24,23)
  Sum1 : Sum  Inputs=|++
  Out1 : Outport
  wires:
  In1/1 -> Sum1/1
  GainH/1 -> Out1/1
  Gain/1 -> Sum1/2
  Delay/1 -> Gain/1
  Sum1/1 -> Delay/1, GainH/1

== system Filter_Fixed/HighpassH/Resonator3 ==
  In1 : Inport
  Delay : Delay  DelayLength=1
  Gain : Gain  Gain=0.67188+0.74066i  OutDataTypeStr=fixdt(1,24,23)
  GainH : Gain  Gain=-0.91984-0.39229i  OutDataTypeStr=fixdt(1,24,23)
  Sum1 : Sum  Inputs=|++
  Out1 : Outport
  wires:
  In1/1 -> Sum1/1
  GainH/1 -> Out1/1
  Gain/1 -> Sum1/2
  Delay/1 -> Gain/1
  Sum1/1 -> Delay/1, GainH/1

== system Filter_Fixed/HighpassH/Resonator30 ==
  In1 : Inport
  Delay : Delay  DelayLength=1
  Gain : Gain  Gain=-0.0139+0.9999i  OutDataTypeStr=fixdt(1,24,23)
  GainH : Gain  Gain=0.712+0.70218i  OutDataTypeStr=fixdt(1,24,23)
  Sum1 : Sum  Inputs=|++
  Out1 : Outport
  wires:
  In1/1 -> Sum1/1
  GainH/1 -> Out1/1
  Gain/1 -> Sum1/2
  Delay/1 -> Gain/1
  Sum1/1 -> Delay/1, GainH/1

== system Filter_Fixed/HighpassH/Resonator31 ==
  In1 : Inport
  Delay : Delay  DelayLength=1
  Gain : Gain  Gain=-0.04169+0.99913i  OutDataTypeStr=fixdt(1,24,23)
  GainH : Gain  Gain=-0.70218-0.712i  OutDataTypeStr=fixdt(1,24,23)
  Sum1 : Sum  Inputs=|++
  Out1 : Outport
  wires:
  In1/1 -> Sum1/1
  GainH/1 -> Out1/1
  Gain/1 -> Sum1/2
  Delay/1 -> Gain/1
  Sum1/1 -> Delay/1, GainH/1

== system Filter_Fixed/HighpassH/Resonator32 ==
  In1 : Inport
  Delay : Delay  DelayLength=1
  Gain : Gain  Gain=-0.069448+0.99759i  OutDataTypeStr=fixdt(1,24,23)
  GainH : Gain  Gain=0.69221+0.7217i  OutDataTypeStr=fixdt(1,24,23)
  Sum1 : Sum  Inputs=|++
  Out1 : Outport
  wires:
  In1/1 -> Sum1/1
  GainH/1 -> Out1/1
  Gain/1 -> Sum1/2
  Delay/1 -> Gain/1
  Sum1/1 -> Delay/1, GainH/1

== system Filter_Fixed/HighpassH/Resonator33 ==
  In1 : Inport
  Delay : Delay  DelayLength=1
  Gain : Gain  Gain=-0.097152+0.99527i  OutDataTypeStr=fixdt(1,24,23)
  GainH : Gain  Gain=-0.68211-0.73125i  OutDataTypeStr=fixdt(1,24,23)
  Sum1 : Sum  Inputs=|++
  Out1 : Outport
  wires:
  In1/1 -> Sum1/1
  GainH/1 -> Out1/1
  Gain/1 -> Sum1/2
  Delay/1 -> Gain/1
  Sum1/1 -> Delay/1, GainH/1

== system Filter_Fixed/HighpassH/Resonator34 ==
  In1 : Inport
  Delay : Delay  DelayLength=1
  Gain : Gain  Gain=-0.12478+0.99218i  OutDataTypeStr=fixdt(1,24,23)
  GainH : Gain  Gain=0.67188+0.74066i  OutDataTypeStr=fixdt(1,24,23)
  Sum1 : Sum  Inputs=|++
  Out1 : Outport
  wires:
  In1/1 -> Sum1/1
  GainH/1 -> Out1/1
  Gain/1 -> Sum1/2
  Delay/1 -> Gain/1
  Sum1/1 -> Delay/1, GainH/1

== system Filter_Fixed/HighpassH/Resonator35 ==
  In1 : Inport
  Delay : Delay  DelayLength=1
  Gain : Gain  Gain=-0.15231+0.98833i  OutDataTypeStr=fixdt(1,24,23)
  GainH : Gain  Gain=-0.66152-0.74993i  OutDataTypeStr=fixdt(1,24,23)
  Sum1 : Sum  Inputs=|++
  Out1 : Outport
  wires:
  In1/1 -> Sum1/1
  GainH/1 -> Out1/1
  Gain/1 -> Sum1/2
  Delay/1 -> Gain/1
  Sum1/1 -> Delay/1, GainH/1

== system Filter_Fixed/HighpassH/Resonator36 ==
  In1 : Inport
  Delay : Delay  DelayLength=1
  Gain : Gain  Gain=-0.17973+0.98372i  OutDataTypeStr=fixdt(1,24,23)
  GainH : Gain  Gain=0.65103+0.75905i  OutDataTypeStr=fixdt(1,24,23)
  Sum1 : Sum  Inputs=|++
  Out1 : Outport
  wires:
  In1/1 -> Sum1/1
  GainH/1 -> Out1/1
  Gain/1 -> Sum1/2
  Delay/1 -> Gain/1
  Sum1/1 -> Delay/1, GainH/1

== system Filter_Fixed/HighpassH/Resonator37 ==
  In1 : Inport
  Delay : Delay  DelayLength=1
  Gain : Gain  Gain=-0.20701+0.97834i  OutDataTypeStr=fixdt(1,24,23)
  GainH : Gain  Gain=-0.64042-0.76803i  OutDataTypeStr=fixdt(1,24,23)
  Sum1 : Sum  Inputs=|++
  Out1 : Outport
  wires:
  In1/1 -> Sum1/1
  GainH/1 -> Out1/1
  Gain/1 -> Sum1/2
  Delay/1 -> Gain/1
  Sum1/1 -> Delay/1, GainH/1

== system Filter_Fixed/HighpassH/Resonator38 ==
  In1 : Inport
  Delay : Delay  DelayLength=1
  Gain : Gain  Gain=-0.23412+0.97221i  OutDataTypeStr=fixdt(1,24,23)
  GainH : Gain  Gain=0.62968+0.77685i  OutDataTypeStr=fixdt(1,24,23)
  Sum1 : Sum  Inputs=|++
  Out1 : Outport
  wires:
  In1/1 -> Sum1/1
  GainH/1 -> Out1/1
  Gain/1 -> Sum1/2
  Delay/1 -> Gain/1
  Sum1/1 -> Delay/1, GainH/1

== system Filter_Fixed/HighpassH/Resonator39 ==
  In1 : Inport
  Delay : Delay  DelayLength=1
  Gain : Gain  Gain=-0.26106+0.96532i  OutDataTypeStr=fixdt(1,24,23)
  GainH : Gain  Gain=-0.61882-0.78553i  OutDataTypeStr=fixdt(1,24,23)
  Sum1 : Sum  Inputs=|++
  Out1 : Outport
  wires:
  In1/1 -> Sum1/1
  GainH/1 -> Out1/1
  Gain/1 -> Sum1/2
  Delay/1 -> Gain/1
  Sum1/1 -> Delay/1, GainH/1

== system Filter_Fixed/HighpassH/Resonator4 ==
  In1 : Inport
  Delay : Delay  DelayLength=1
  Gain : Gain  Gain=0.65103+0.75905i  OutDataTypeStr=fixdt(1,24,23)
  GainH : Gain  Gain=0.9143+0.40504i  OutDataTypeStr=fixdt(1,24,23)
  Sum1 : Sum  Inputs=|++
  Out1 : Outport
  wires:
  In1/1 -> Sum1/1
  GainH/1 -> Out1/1
  Gain/1 -> Sum1/2
  Delay/1 -> Gain/1
  Sum1/1 -> Delay/1, GainH/1

== system Filter_Fixed/HighpassH/Resonator40 ==
  In1 : Inport
  Delay : Delay  DelayLength=1
  Gain : Gain  Gain=-0.28779+0.95769i  OutDataTypeStr=fixdt(1,24,23)
  GainH : Gain  Gain=0.60784+0.79406i  OutDataTypeStr=fixdt(1,24,23)
  Sum1 : Sum  Inputs=|++
  Out1 : Outport
  wires:
  In1/1 -> Sum1/1
  GainH/1 -> Out1/1
  Gain/1 -> Sum1/2
  Delay/1 -> Gain/1
  Sum1/1 -> Delay/1, GainH/1

== system Filter_Fixed/HighpassH/Resonator41 ==
  In1 : Inport
  Delay : Delay  DelayLength=1
  Gain : Gain  Gain=-0.3143+0.94932i  OutDataTypeStr=fixdt(1,24,23)
  GainH : Gain  Gain=-0.59675-0.80243i  OutDataTypeStr=fixdt(1,24,23)
  Sum1 : Sum  Inputs=|++
  Out1 : Outport
  wires:
  In1/1 -> Sum1/1
  GainH/1 -> Out1/1
  Gain/1 -> Sum1/2
  Delay/1 -> Gain/1
  Sum1/1 -> Delay/1, GainH/1

== system Filter_Fixed/HighpassH/Resonator42 ==
  In1 : Inport
  Delay : Delay  DelayLength=1
  Gain : Gain  Gain=-0.34057+0.94022i  OutDataTypeStr=fixdt(1,24,23)
  GainH : Gain  Gain=0.58553+0.81065i  OutDataTypeStr=fixdt(1,24,23)
  Sum1 : Sum  Inputs=|++
  Out1 : Outport
  wires:
  In1/1 -> Sum1/1
  GainH/1 -> Out1/1
  Gain/1 -> Sum1/2
  Delay/1 -> Gain/1
  Sum1/1 -> Delay/1, GainH/1

== system Filter_Fixed/HighpassH/Resonator43 ==
  In1 : Inport
  Delay : Delay  DelayLength=1
  Gain : Gain  Gain=-0.36657+0.93039i  OutDataTypeStr=fixdt(1,24,23)
  GainH : Gain  Gain=-0.57421-0.81871i  OutDataTypeStr=fixdt(1,24,23)
  Sum1 : Sum  Inputs=|++
  Out1 : Outport
  wires:
  In1/1 -> Sum1/1
  GainH/1 -> Out1/1
  Gain/1 -> Sum1/2
  Delay/1 -> Gain/1
  Sum1/1 -> Delay/1, GainH/1

== system Filter_Fixed/HighpassH/Resonator44 ==
  In1 : Inport
  Delay : Delay  DelayLength=1
  Gain : Gain  Gain=-0.39229+0.91984i  OutDataTypeStr=fixdt(1,24,23)
  GainH : Gain  Gain=0.56277+0.82661i  OutDataTypeStr=fixdt(1,24,23)
  Sum1 : Sum  Inputs=|++
  Out1 : Outport
  wires:
  In1/1 -> Sum1/1
  GainH/1 -> Out1/1
  Gain/1 -> Sum1/2
  Delay/1 -> Gain/1
  Sum1/1 -> Delay/1, GainH/1

== system Filter_Fixed/HighpassH/Resonator45 ==
  In1 : Inport
  Delay : Delay  DelayLength=1
  Gain : Gain  Gain=-0.41771+0.90858i  OutDataTypeStr=fixdt(1,24,23)
  GainH : Gain  Gain=-0.55123-0.83435i  OutDataTypeStr=fixdt(1,24,23)
  Sum1 : Sum  Inputs=|++
  Out1 : Outport
  wires:
  In1/1 -> Sum1/1
  GainH/1 -> Out1/1
  Gain/1 -> Sum1/2
  Delay/1 -> Gain/1
  Sum1/1 -> Delay/1, GainH/1

== system Filter_Fixed/HighpassH/Resonator46 ==
  In1 : Inport
  Delay : Delay  DelayLength=1
  Gain : Gain  Gain=-0.44281+0.89662i  OutDataTypeStr=fixdt(1,24,23)
  GainH : Gain  Gain=0.53958+0.84194i  OutDataTypeStr=fixdt(1,24,23)
  Sum1 : Sum  Inputs=|++
  Out1 : Outport
  wires:
  In1/1 -> Sum1/1
  GainH/1 -> Out1/1
  Gain/1 -> Sum1/2
  Delay/1 -> Gain/1
  Sum1/1 -> Delay/1, GainH/1

== system Filter_Fixed/HighpassH/Resonator47 ==
  In1 : Inport
  Delay : Delay  DelayLength=1
  Gain : Gain  Gain=-0.46756+0.88396i  OutDataTypeStr=fixdt(1,24,23)
  GainH : Gain  Gain=-0.52782-0.84936i  OutDataTypeStr=fixdt(1,24,23)
  Sum1 : Sum  Inputs=|++
  Out1 : Outport
  wires:
  In1/1 -> Sum1/1
  GainH/1 -> Out1/1
  Gain/1 -> Sum1/2
  Delay/1 -> Gain/1
  Sum1/1 -> Delay/1, GainH/1

== system Filter_Fixed/HighpassH/Resonator48 ==
  In1 : Inport
  Delay : Delay  DelayLength=1
  Gain : Gain  Gain=-0.49195+0.87062i  OutDataTypeStr=fixdt(1,24,23)
  GainH : Gain  Gain=0.51596+0.85661i  OutDataTypeStr=fixdt(1,24,23)
  Sum1 : Sum  Inputs=|++
  Out1 : Outport
  wires:
  In1/1 -> Sum1/1
  GainH/1 -> Out1/1
  Gain/1 -> Sum1/2
  Delay/1 -> Gain/1
  Sum1/1 -> Delay/1, GainH/1

== system Filter_Fixed/HighpassH/Resonator49 ==
  In1 : Inport
  Delay : Delay  DelayLength=1
  Gain : Gain  Gain=-0.51596+0.85661i  OutDataTypeStr=fixdt(1,24,23)
  GainH : Gain  Gain=-0.50401-0.8637i  OutDataTypeStr=fixdt(1,24,23)
  Sum1 : Sum  Inputs=|++
  Out1 : Outport
  wires:
  In1/1 -> Sum1/1
  GainH/1 -> Out1/1
  Gain/1 -> Sum1/2
  Delay/1 -> Gain/1
  Sum1/1 -> Delay/1, GainH/1

== system Filter_Fixed/HighpassH/Resonator5 ==
  In1 : Inport
  Delay : Delay  DelayLength=1
  Gain : Gain  Gain=0.62968+0.77685i  OutDataTypeStr=fixdt(1,24,23)
  GainH : Gain  Gain=-0.90858-0.41771i  OutDataTypeStr=fixdt(1,24,23)
  Sum1 : Sum  Inputs=|++
  Out1 : Outport
  wires:
  In1/1 -> Sum1/1
  GainH/1 -> Out1/1
  Gain/1 -> Sum1/2
  Delay/1 -> Gain/1
  Sum1/1 -> Delay/1, GainH/1

== system Filter_Fixed/HighpassH/Resonator50 ==
  In1 : Inport
  Delay : Delay  DelayLength=1
  Gain : Gain  Gain=-0.53958+0.84194i  OutDataTypeStr=fixdt(1,24,23)
  GainH : Gain  Gain=0.49195+0.87062i  OutDataTypeStr=fixdt(1,24,23)
  Sum1 : Sum  Inputs=|++
  Out1 : Outport
  wires:
  In1/1 -> Sum1/1
  GainH/1 -> Out1/1
  Gain/1 -> Sum1/2
  Delay/1 -> Gain/1
  Sum1/1 -> Delay/1, GainH/1

== system Filter_Fixed/HighpassH/Resonator51 ==
  In1 : Inport
  Delay : Delay  DelayLength=1
  Gain : Gain  Gain=-0.56277+0.82661i  OutDataTypeStr=fixdt(1,24,23)
  GainH : Gain  Gain=-0.4798-0.87738i  OutDataTypeStr=fixdt(1,24,23)
  Sum1 : Sum  Inputs=|++
  Out1 : Outport
  wires:
  In1/1 -> Sum1/1
  GainH/1 -> Out1/1
  Gain/1 -> Sum1/2
  Delay/1 -> Gain/1
  Sum1/1 -> Delay/1, GainH/1

== system Filter_Fixed/HighpassH/Resonator52 ==
  In1 : Inport
  Delay : Delay  DelayLength=1
  Gain : Gain  Gain=-0.58553+0.81065i  OutDataTypeStr=fixdt(1,24,23)
  GainH : Gain  Gain=0.46756+0.88396i  OutDataTypeStr=fixdt(1,24,23)
  Sum1 : Sum  Inputs=|++
  Out1 : Outport
  wires:
  In1/1 -> Sum1/1
  GainH/1 -> Out1/1
  Gain/1 -> Sum1/2
  Delay/1 -> Gain/1
  Sum1/1 -> Delay/1, GainH/1

== system Filter_Fixed/HighpassH/Resonator53 ==
  In1 : Inport
  Delay : Delay  DelayLength=1
  Gain : Gain  Gain=-0.60784+0.79406i  OutDataTypeStr=fixdt(1,24,23)
  GainH : Gain  Gain=-0.45523-0.89037i  OutDataTypeStr=fixdt(1,24,23)
  Sum1 : Sum  Inputs=|++
  Out1 : Outport
  wires:
  In1/1 -> Sum1/1
  GainH/1 -> Out1/1
  Gain/1 -> Sum1/2
  Delay/1 -> Gain/1
  Sum1/1 -> Delay/1, GainH/1

== system Filter_Fixed/HighpassH/Resonator54 ==
  In1 : Inport
  Delay : Delay  DelayLength=1
  Gain : Gain  Gain=-0.62968+0.77685i  OutDataTypeStr=fixdt(1,24,23)
  GainH : Gain  Gain=0.44281+0.89662i  OutDataTypeStr=fixdt(1,24,23)
  Sum1 : Sum  Inputs=|++
  Out1 : Outport
  wires:
  In1/1 -> Sum1/1
  GainH/1 -> Out1/1
  Gain/1 -> Sum1/2
  Delay/1 -> Gain/1
  Sum1/1 -> Delay/1, GainH/1

== system Filter_Fixed/HighpassH/Resonator55 ==
  In1 : Inport
  Delay : Delay  DelayLength=1
  Gain : Gain  Gain=-0.65103+0.75905i  OutDataTypeStr=fixdt(1,24,23)
  GainH : Gain  Gain=-0.4303-0.90269i  OutDataTypeStr=fixdt(1,24,23)
  Sum1 : Sum  Inputs=|++
  Out1 : Outport
  wires:
  In1/1 -> Sum1/1
  GainH/1 -> Out1/1
  Gain/1 -> Sum1/2
  Delay/1 -> Gain/1
  Sum1/1 -> Delay/1, GainH/1

== system Filter_Fixed/HighpassH/Resonator56 ==
  In1 : Inport
  Delay : Delay  DelayLength=1
  Gain : Gain  Gain=-0.67188+0.74066i  OutDataTypeStr=fixdt(1,24,23)
  GainH : Gain  Gain=0.41771+0.90858i  OutDataTypeStr=fixdt(1,24,23)
  Sum1 : Sum  Inputs=|++
  Out1 : Outport
  wires:
  In1/1 -> Sum1/1
  GainH/1 -> Out1/1
  Gain/1 -> Sum1/2
  Delay/1 -> Gain/1
  Sum1/1 -> Delay/1, GainH/1

== system Filter_Fixed/HighpassH/Resonator57 ==
  In1 : Inport
  Delay : Delay  DelayLength=1
  Gain : Gain  Gain=-0.69221+0.7217i  OutDataTypeStr=fixdt(1,24,23)
  GainH : Gain  Gain=-0.40504-0.9143i  OutDataTypeStr=fixdt(1,24,23)
  Sum1 : Sum  Inputs=|++
  Out1 : Outport
  wires:
  In1/1 -> Sum1/1
  GainH/1 -> Out1/1
  Gain/1 -> Sum1/2
  Delay/1 -> Gain/1
  Sum1/1 -> Delay/1, GainH/1

== system Filter_Fixed/HighpassH/Resonator58 ==
  In1 : Inport
  Delay : Delay  DelayLength=1
  Gain : Gain  Gain=-0.712+0.70218i  OutDataTypeStr=fixdt(1,24,23)
  GainH : Gain  Gain=0.39229+0.91984i  OutDataTypeStr=fixdt(1,24,23)
  Sum1 : Sum  Inputs=|++
  Out1 : Outport
  wires:
  In1/1 -> Sum1/1
  GainH/1 -> Out1/1
  Gain/1 -> Sum1/2
  Delay/1 -> Gain/1
  Sum1/1 -> Delay/1, GainH/1

== system Filter_Fixed/HighpassH/Resonator59 ==
  In1 : Inport
  Delay : Delay  DelayLength=1
  Gain : Gain  Gain=-0.73125+0.68211i  OutDataTypeStr=fixdt(1,24,23)
  GainH : Gain  Gain=-0.37947-0.9252i  OutDataTypeStr=fixdt(1,24,23)
  Sum1 : Sum  Inputs=|++
  Out1 : Outport
  wires:
  In1/1 -> Sum1/1
  GainH/1 -> Out1/1
  Gain/1 -> Sum1/2
  Delay/1 -> Gain/1
  Sum1/1 -> Delay/1, GainH/1

== system Filter_Fixed/HighpassH/Resonator6 ==
  In1 : Inport
  Delay : Delay  DelayLength=1
  Gain : Gain  Gain=0.60784+0.79406i  OutDataTypeStr=fixdt(1,24,23)
  GainH : Gain  Gain=0.90269+0.4303i  OutDataTypeStr=fixdt(1,24,23)
  Sum1 : Sum  Inputs=|++
  Out1 : Outport
  wires:
  In1/1 -> Sum1/1
  GainH/1 -> Out1/1
  Gain/1 -> Sum1/2
  Delay/1 -> Gain/1
  Sum1/1 -> Delay/1, GainH/1

== system Filter_Fixed/HighpassH/Resonator60 ==
  In1 : Inport
  Delay : Delay  DelayLength=1
  Gain : Gain  Gain=-0.74993+0.66152i  OutDataTypeStr=fixdt(1,24,23)
  GainH : Gain  Gain=0.36657+0.93039i  OutDataTypeStr=fixdt(1,24,23)
  Sum1 : Sum  Inputs=|++
  Out1 : Outport
  wires:
  In1/1 -> Sum1/1
  GainH/1 -> Out1/1
  Gain/1 -> Sum1/2
  Delay/1 -> Gain/1
  Sum1/1 -> Delay/1, GainH/1

== system Filter_Fixed/HighpassH/Resonator61 ==
  In1 : Inport
  Delay : Delay  DelayLength=1
  Gain : Gain  Gain=-0.76803+0.64042i  OutDataTypeStr=fixdt(1,24,23)
  GainH : Gain  Gain=-0.3536-0.93539i  OutDataTypeStr=fixdt(1,24,23)
  Sum1 : Sum  Inputs=|++
  Out1 : Outport
  wires:
  In1/1 -> Sum1/1
  GainH/1 -> Out1/1
  Gain/1 -> Sum1/2
  Delay/1 -> Gain/1
  Sum1/1 -> Delay/1, GainH/1

== system Filter_Fixed/HighpassH/Resonator62 ==
  In1 : Inport
  Delay : Delay  DelayLength=1
  Gain : Gain  Gain=-0.78553+0.61882i  OutDataTypeStr=fixdt(1,24,23)
  GainH : Gain  Gain=0.34057+0.94022i  OutDataTypeStr=fixdt(1,24,23)
  Sum1 : Sum  Inputs=|++
  Out1 : Outport
  wires:
  In1/1 -> Sum1/1
  GainH/1 -> Out1/1
  Gain/1 -> Sum1/2
  Delay/1 -> Gain/1
  Sum1/1 -> Delay/1, GainH/1

== system Filter_Fixed/HighpassH/Resonator63 ==
  In1 : Inport
  Delay : Delay  DelayLength=1
  Gain : Gain  Gain=-0.80243+0.59675i  OutDataTypeStr=fixdt(1,24,23)
  GainH : Gain  Gain=-0.32747-0.94486i  OutDataTypeStr=fixdt(1,24,23)
  Sum1 : Sum  Inputs=|++
  Out1 : Outport
  wires:
  In1/1 -> Sum1/1
  GainH/1 -> Out1/1
  Gain/1 -> Sum1/2
  Delay/1 -> Gain/1
  Sum1/1 -> Delay/1, GainH/1

== system Filter_Fixed/HighpassH/Resonator64 ==
  In1 : Inport
  Delay : Delay  DelayLength=1
  Gain : Gain  Gain=-0.81871+0.57421i  OutDataTypeStr=fixdt(1,24,23)
  GainH : Gain  Gain=0.3143+0.94932i  OutDataTypeStr=fixdt(1,24,23)
  Sum1 : Sum  Inputs=|++
  Out1 : Outport
  wires:
  In1/1 -> Sum1/1
  GainH/1 -> Out1/1
  Gain/1 -> Sum1/2
  Delay/1 -> Gain/1
  Sum1/1 -> Delay/1, GainH/1

== system Filter_Fixed/HighpassH/Resonator65 ==
  In1 : Inport
  Delay : Delay  DelayLength=1
  Gain : Gain  Gain=-0.83435+0.55123i  OutDataTypeStr=fixdt(1,24,23)
  GainH : Gain  Gain=-0.30107-0.9536i  OutDataTypeStr=fixdt(1,24,23)
  Sum1 : Sum  Inputs=|++
  Out1 : Outport
  wires:
  In1/1 -> Sum1/1
  GainH/1 -> Out1/1
  Gain/1 -> Sum1/2
  Delay/1 -> Gain/1
  Sum1/1 -> Delay/1, GainH/1

== system Filter_Fixed/HighpassH/Resonator66 ==
  In1 : Inport
  Delay : Delay  DelayLength=1
  Gain : Gain  Gain=-0.84936+0.52782i  OutDataTypeStr=fixdt(1,24,23)
  GainH : Gain  Gain=0.28779+0.95769i  OutDataTypeStr=fixdt(1,24,23)
  Sum1 : Sum  Inputs=|++
  Out1 : Outport
  wires:
  In1/1 -> Sum1/1
  GainH/1 -> Out1/1
  Gain/1 -> Sum1/2
  Delay/1 -> Gain/1
  Sum1/1 -> Delay/1, GainH/1

== system Filter_Fixed/HighpassH/Resonator67 ==
  In1 : Inport
  Delay : Delay  DelayLength=1
  Gain : Gain  Gain=-0.8637+0.50401i  OutDataTypeStr=fixdt(1,24,23)
  GainH : Gain  Gain=-0.27445-0.9616i  OutDataTypeStr=fixdt(1,24,23)
  Sum1 : Sum  Inputs=|++
  Out1 : Outport
  wires:
  In1/1 -> Sum1/1
  GainH/1 -> Out1/1
  Gain/1 -> Sum1/2
  Delay/1 -> Gain/1
  Sum1/1 -> Delay/1, GainH/1

== system Filter_Fixed/HighpassH/Resonator68 ==
  In1 : Inport
  Delay : Delay  DelayLength=1
  Gain : Gain  Gain=-0.87738+0.4798i  OutDataTypeStr=fixdt(1,24,23)
  GainH : Gain  Gain=0.26106+0.96532i  OutDataTypeStr=fixdt(1,24,23)
  Sum1 : Sum  Inputs=|++
  Out1 : Outport
  wires:
  In1/1 -> Sum1/1
  GainH/1 -> Out1/1
  Gain/1 -> Sum1/2
  Delay/1 -> Gain/1
  Sum1/1 -> Delay/1, GainH/1

== system Filter_Fixed/HighpassH/Resonator69 ==
  In1 : Inport
  Delay : Delay  DelayLength=1
  Gain : Gain  Gain=-0.89037+0.45523i  OutDataTypeStr=fixdt(1,24,23)
  GainH : Gain  Gain=-0.24761-0.96886i  OutDataTypeStr=fixdt(1,24,23)
  Sum1 : Sum  Inputs=|++
  Out1 : Outport
  wires:
  In1/1 -> Sum1/1
  GainH/1 -> Out1/1
  Gain/1 -> Sum1/2
  Delay/1 -> Gain/1
  Sum1/1 -> Delay/1, GainH/1

== system Filter_Fixed/HighpassH/Resonator7 ==
  In1 : Inport
  Delay : Delay  DelayLength=1
  Gain : Gain  Gain=0.58553+0.81065i  OutDataTypeStr=fixdt(1,24,23)
  GainH : Gain  Gain=-0.89662-0.44281i  OutDataTypeStr=fixdt(1,24,23)
  Sum1 : Sum  Inputs=|++
  Out1 : Outport
  wires:
  In1/1 -> Sum1/1
  GainH/1 -> Out1/1
  Gain/1 -> Sum1/2
  Delay/1 -> Gain/1
  Sum1/1 -> Delay/1, GainH/1

== system Filter_Fixed/HighpassH/Resonator70 ==
  In1 : Inport
  Delay : Delay  DelayLength=1
  Gain : Gain  Gain=-0.90269+0.4303i  OutDataTypeStr=fixdt(1,24,23)
  GainH : Gain  Gain=0.23412+0.97221i  OutDataTypeStr=fixdt(1,24,23)
  Sum1 : Sum  Inputs=|++
  Out1 : Outport
  wires:
  In1/1 -> Sum1/1
  GainH/1 -> Out1/1
  Gain/1 -> Sum1/2
  Delay/1 -> Gain/1
  Sum1/1 -> Delay/1, GainH/1

== system Filter_Fixed/HighpassH/Resonator71 ==
  In1 : Inport
  Delay : Delay  DelayLength=1
  Gain : Gain  Gain=-0.9143+0.40504i  OutDataTypeStr=fixdt(1,24,23)
  GainH : Gain  Gain=-0.22058-0.97537i  OutDataTypeStr=fixdt(1,24,23)
  Sum1 : Sum  Inputs=|++
  Out1 : Outport
  wires:
  In1/1 -> Sum1/1
  GainH/1 -> Out1/1
  Gain/1 -> Sum1/2
  Delay/1 -> Gain/1
  Sum1/1 -> Delay/1, GainH/1

== system Filter_Fixed/HighpassH/Resonator72 ==
  In1 : Inport
  Delay : Delay  DelayLength=1
  Gain : Gain  Gain=-0.9252+0.37947i  OutDataTypeStr=fixdt(1,24,23)
  GainH : Gain  Gain=0.20701+0.97834i  OutDataTypeStr=fixdt(1,24,23)
  Sum1 : Sum  Inputs=|++
  Out1 : Outport
  wires:
  In1/1 -> Sum1/1
  GainH/1 -> Out1/1
  Gain/1 -> Sum1/2
  Delay/1 -> Gain/1
  Sum1/1 -> Delay/1, GainH/1

== system Filter_Fixed/HighpassH/Resonator73 ==
  In1 : Inport
  Delay : Delay  DelayLength=1
  Gain : Gain  Gain=-0.93539+0.3536i  OutDataTypeStr=fixdt(1,24,23)
  GainH : Gain  Gain=-0.19339-0.98112i  OutDataTypeStr=fixdt(1,24,23)
  Sum1 : Sum  Inputs=|++
  Out1 : Outport
  wires:
  In1/1 -> Sum1/1
  GainH/1 -> Out1/1
  Gain/1 -> Sum1/2
  Delay/1 -> Gain/1
  Sum1/1 -> Delay/1, GainH/1

== system Filter_Fixed/HighpassH/Resonator74 ==
  In1 : Inport
  Delay : Delay  DelayLength=1
  Gain : Gain  Gain=-0.94486+0.32747i  OutDataTypeStr=fixdt(1,24,23)
  GainH : Gain  Gain=0.17973+0.98372i  OutDataTypeStr=fixdt(1,24,23)
  Sum1 : Sum  Inputs=|++
  Out1 : Outport
  wires:
  In1/1 -> Sum1/1
  GainH/1 -> Out1/1
  Gain/1 -> Sum1/2
  Delay/1 -> Gain/1
  Sum1/1 -> Delay/1, GainH/1
